simulink model "CONTROL_SYSTEM_V3"  (R2024a)
settings: Solver=FixedStepAuto  StartTime=0.0  StopTime=inf  FixedStep=0.01  RelTol=1e-3
values from neighbouring files (symbols this model uses):
  Beta1 = 3*Omega_o    (= 15)    [CONTROL_SYSTEM_VAR.m]
  Beta2 = 3*(Omega_o^2)    (= 75)    [CONTROL_SYSTEM_VAR.m]
  Beta3 = (Omega_o^3)    (= 125)    [CONTROL_SYSTEM_VAR.m]
  Desire_Max = 255    [CONTROL_SYSTEM_VAR.m]
  Desire_Min = 0    [CONTROL_SYSTEM_VAR.m]
  Direction_Pin = 1    [CONTROL_SYSTEM_VAR.m]
  EN_Pin = 0    [CONTROL_SYSTEM_VAR.m]
  J_aet = 0.0035    [CONTROL_SYSTEM_VAR.m]
  Kd = 2    [CONTROL_SYSTEM_VAR.m]
  Ki = 4    [CONTROL_SYSTEM_VAR.m]
  Kn = 0.1    [CONTROL_SYSTEM_VAR.m]
  Kp = 1.4    [CONTROL_SYSTEM_VAR.m]
  omga_c = 10    [CONTROL_SYSTEM_VAR.m]
  roa = 0.24    [CONTROL_SYSTEM_VAR.m]
undefined symbols (not defined in the file or in its folder): sigbuilder_block
libraries: arduinolib x30, simulink_extras x14, simulink x5, slpidlib x4, SignalEditorBlockLib x3, slctrl_adaptive x2, spsOnDelayLib x2, slctrl_autotuning x2
(part 2 of 5)

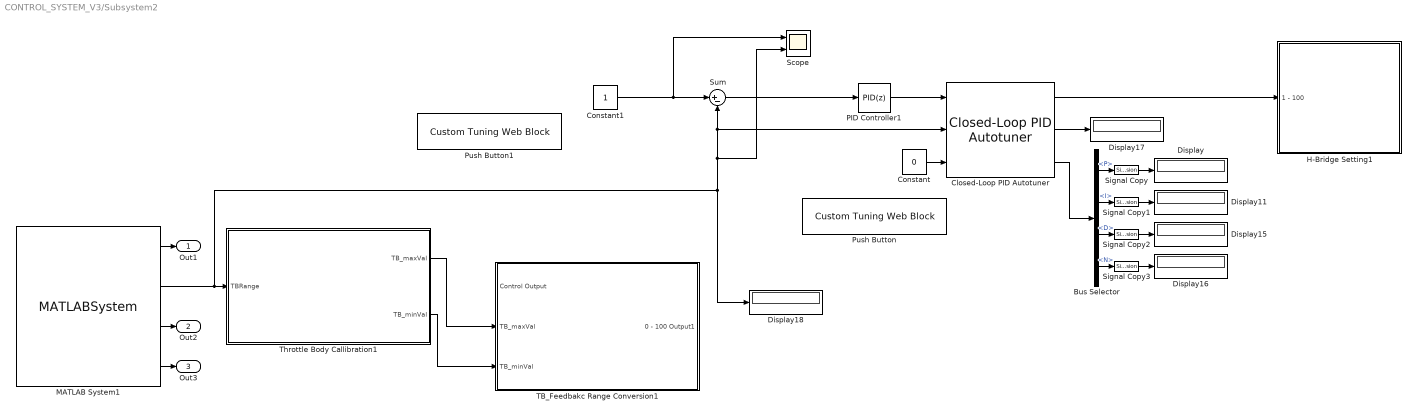
== system CONTROL_SYSTEM_V3/Subsystem2 ==
  Bus Selector : BusSelector  OutputSignals=P,I,D,N
  Closed-Loop PID Autotuner : slctrl_autotuning/Closed-Loop PID Autotuner  PIDType=PID  PIDForm=Parallel  TimeDomain=discrete-time  DiscreteTs=0.1  TuningTs=0.2  UseTuningTs=off  IntegratorFormula=Forward Euler  FilterFormula=Forward Euler  ContinuousTs=-1  Bandwidth=1  UseExternalWC=off  TargetPM=60  UseExternalPM=off  UseExternalAchievedPM=off  ExperimentMode=Superposition  PlantType=Stable  PlantSign=Positive  AmpSine=1  UseExternalAmpSine=off  UseExternalFRD=off  UseExternalU0=off  UseCompanion=off  NotDeployTuningModule=off  UsePLCCoder=off  OutputMode=control action + perturbation  BlockDataType=double  UseConnectedPID=on  blockpath=[]  tunedP=0  tunedI=0  tunedD=0  tunedN=100  tunedPM=0  EstimationWindowSize=3  UseExternalTuningParams=off  SingleMultiRateVariant=SingleSamplingRate  NumEstimationPeriods=4  NumSettlingPeriods=2  NumOfPRBSPeriod=1  PRBSSignalOrder=12  ExperimentModeVariant=VariantSuperimposed  OutputChoice=VariantCandD
      settings: LibrarySourceBlock=slctrlblks/Autotuning/Closed-Loop PID Autotuner
  Constant : Constant  Value=0
  Constant1 : Constant
  Display{,11,15..18} (6 alike) : Display
  H-Bridge Setting1 : Subsystem
      mask Display: image('H-Bridge.JPG');
  MATLAB System1 : MATLABSystem  System=ADS1115_Vread  SetGain=int16( 16 )  SampleTime=-1
      mask Type: ADS1115_Vread
      mask Display:
      | color('white');plot([100,100,100,100]*1,[100,100,100,100]*1);plot([100,100,100,100]*0,[100,100,100,100]*0);color('blue');text(38, 92, 'IO Device Builder','horizontalAlignment', 'right');
      | color('black');text(52,50,' ADS1115_Vread','horizontalAlignment','center');
      | port_label('output',1,'V0');port_label('output',2,'V1');port_label('output',3,'V2');port_label('output',4,'V3');
  PID Controller1 : slpidlib/PID Controller  Controller=PID  Form=Parallel  TimeDomain=Discrete-time  UseExternalTs=off  SampleTime=-1  IntegratorMethod=Forward Euler  FilterMethod=Forward Euler  ControllerParametersSource=internal  P=0  I=185.8371  UseKiTs=off  D=87.2762  UseExternalDerivativeSource=off  N=100  UseFilter=on  TunerSelectOption=Transfer Function Based (PID Tuner App)  InitialConditionSource=internal  InitialConditionForIntegrator=0  InitialConditionForFilter=0  DifferentiatorICPrevScaledInput=0  ExternalReset=none  TrackingMode=off  Kt=1  LimitOutput=off  SatLimitsSource=internal  UpperSaturationLimit=inf  LowerSaturationLimit=-inf  LinearizeAsGain=on  AntiWindupMode=none  Kb=1  LimitIntegrator=off  UpperIntegratorSaturationLimit=inf  LowerIntegratorSaturationLimit=-inf  POutMin=[]  POutMax=[]  IOutMin=[]  IOutMax=[]  DOutMin=[]  DOutMax=[]  NOutMin=[]  NOutMax=[]  SumOutMin=[]  SumOutMax=[]  SaturationOutMin=[]  SaturationOutMax=[]  PParamMin=[]  PParamMax=[]  IParamMin=[]  IParamMax=[]  DParamMin=[]  DParamMax=[]  NParamMin=[]  NParamMax=[]  KbParamMin=[]  KbParamMax=[]  KtParamMin=[]  KtParamMax=[]  KbOutMin=[]  KbOutMax=[]  KtOutMin=[]  KtOutMax=[]  IntegratorOutMin=[]  IntegratorOutMax=[]  FilterOutMin=[]  FilterOutMax=[]  SumI1OutMin=[]  SumI1OutMax=[]  SumI2OutMin=[]  SumI2OutMax=[]  SumI3OutMin=[]  SumI3OutMax=[]  SumI4OutMin=[]  SumI4OutMax=[]  SumDOutMin=[]  SumDOutMax=[]  DifferentiatorOutMin=[]  DifferentiatorOutMax=[]  FilterDiffOutCoefMin=[]  FilterDiffOutCoefMax=[]  ReciprocalOutMin=[]  ReciprocalOutMax=[]  SumDenOutMin=[]  SumDenOutMax=[]  SumNumOutMin=[]  SumNumOutMax=[]  DivideOutMin=[]  DivideOutMax=[]  UdiffTsProdOutMin=[]  UdiffTsProdOutMax=[]  NTsProdOutMin=[]  NTsProdOutMax=[]  UintegralTsProdOutMin=[]  UintegralTsProdOutMax=[]  UngainTsProdOutMin=[]  UngainTsProdOutMax=[]  ClampingZeroOutDataTypeStr=Inherit: Inherit via back propagation  ClampingZeroOutMin=[]  ClampingZeroOutMax=[]  FilterDenConstantOutDataTypeStr=Inherit: Inherit via back propagation  FilterDenConstantOutMin=[]  FilterDenConstantOutMax=[]  PCopyOutDataTypeStr=Inherit: Inherit via back propagation  PCopyOutMin=[]  PCopyOutMax=[]  NCopyOutDataTypeStr=Inherit: Inherit via back propagation  NCopyOutMin=[]  NCopyOutMax=[]  IntegratorContinuousStateAttributes=''  IntegratorStateMustResolveToSignalObject=off  IntegratorRTWStateStorageClass=Auto  FilterContinuousStateAttributes=''  FilterStateMustResolveToSignalObject=off  FilterRTWStateStorageClass=Auto  ParallelPVariant=InternalParameters  IdealPVariant=Disabled  IVariant=InternalParameters  DVariant=InternalParameters  IntegratorVariant=Discrete  SatVariant=Disabled  AWVariant=Passthrough  PCopyVariant=Disabled  TRVariant=Disabled  FdbkBlocksVariant=Forward  IdealPFdbkVariant=Disabled  SatFdbkVariant=Disabled  DerivativeFilterVariant=ForwardEulerFilter  NVariant=InternalParameters  NCopyVariant=Disabled  FilterICVariant=InternalICsFilter  IntegratorICVariant=InternalICs  ExternalResetVariant=Disabled  TRSumVariant=Passthrough  SumFdbkVariant=Disabled  SumVariant=Sum_PID  TsampFilterVariant=InternalTs  TsampNgainVariant=Passthrough  TsampIntegralVariant=Disabled_SignalSpec  ExternalSaturationOutDataTypeStr=Inherit: Same as second input  DerivativeSourceVariant=ErrorSignal
  Push Button : CustomTuningWebBlock  LabelPosition=Hide  ShowInitialText=on  Configuration="{\"components\":[{\"name\":\"BackgroundImageComponent\",\"settings\":{\"image\":{\"size\":[0,0],\"src\":\"default\",\"srcOrientation\":\"horizontal\"},\"position\":[0,0,1,1],\"scaleMode\":\"0\"}},{\"name\":\"ButtonStateComponent\",\"settings\":{\"buttonType\":\"latch\",\"clickFcn\":\"\",\"image\":{\"size\":[180,45],\"srcOrientation\":\"Right\"},\"latched\":false,\"offValue\":null,\"onValue\":\"1\",\"position\":[0,0,1,1],\"pressDelay\":\"500\",\"pressFcn\":\"\",\"repeatInterval\":\"0\",\"states\":[{\"horizontalAlignment\":\"center\",\"image\":{\"position\":[0.04444444444444445,0.005555555555555536,0.9888888888888889,0.9111111111111111],\"size\":[0.9888888888888889,0.9111111111111111],\"src\":\"data:image\\/svg+xml;base64,PHN2ZyB4bWxucz0iaHR0cDovL3d3dy53My5vcmcvMjAwMC9zdmciIHhtbG5zOnhsaW5rPSJodHRwOi8vd3d3LnczLm9yZy8xOTk5L3hsaW5rIiB2aWV3Qm94PSIwIDAgMTc3LjI1IDQwLjg4Ij48ZGVmcz48c3R5bGU+LmNscy0xe2ZpbGw6dXJsKCNyYWRpYWwtZ3JhZGllbnQpO30uY2xzLTJ7ZmlsbDp1cmwoI2xpbmVhci1ncmFkaWVudCk7fS5jbHMtM3tmaWxsOnVybCgjbGluZWFyLWdyYWRpZW50LTIpO308L3N0eWxlPjxyYWRpYWxHcmFkaWVudCBpZD0icmFkaWFsLWdyYWRpZW50IiBjeD0iOTAuMDkiIGN5PSIyMi42NiIgcj0i ...(+2212 chars)\",\"srcOrientation\":\"Right\"},\"label\":{\"color\":[1,1,0.78,1],\"icon\":{\"size\":[0.1,0.375],\"src\":\"data:image\\/svg+xml;base64,PHN2ZyBpZD0iT2ZmIiB4bWxucz0iaHR0cDovL3d3dy53My5vcmcvMjAwMC9zdmciIHhtbG5zOnhsaW5rPSJodHRwOi8vd3d3LnczLm9yZy8xOTk5L3hsaW5rIiB2aWV3Qm94PSIwIDAgNTAgNTAiPjxkZWZzPjxzdHlsZT4uY2xzLTF7ZmlsbDojN2Y4MDgwO3N0cm9rZTojMjcyNjI2O3N0cm9rZS1taXRlcmxpbWl0OjEwO3N0cm9rZS13aWR0aDozcHg7fS5jbHMtMntmaWxsOnVybCgjbGluZWFyLWdyYWRpZW50KTt9PC9zdHlsZT48bGluZWFyR3JhZGllbnQgaWQ9ImxpbmVhci1ncmFkaWVudCIgeDE9IjI1IiB5MT0iOSIgeDI9IjI1IiB5Mj0iMzciIGdyYWRpZW50VW5pdHM9InVzZXJTcGFjZU9uVXNlIj48c3RvcCBvZmZzZXQ9IjAiIHN0b3AtY29sb3I9IiNmZmYiIHN0b3Atb3BhY2l0eT0iMC43NSIvPjxzdG9wIG9mZnNldD0iMSIgc3RvcC1jb2xvcj0iI2ZmZiIgc3RvcC1vcGFjaXR5PSIwIi8+PC9saW5lYXJHcmFkaWVudD48L2RlZnM+PGNpcmNsZSBjbGFzcz0iY2xzLTEiIGN4PSIyNSIgY3k9IjI1IiByPSIyMCIvPjxjaXJjbGUgY2xhc3M9ImNscy0yIiBjeD0iMjUiIGN5PSIyMyIgcj0iMTQiLz48L3N2Zz4=\",\"srcOrientation\":\"Right\"},\"iconPlacement\":\"left\",\"opacity\":1,\"show\":true,\"text\":{\"content\":\"Button\",\"font\":\"Helvetica\",\"fontSize\":14}},\"labelOffset\":[0,0],\"verticalAlignment\":\"middle\"},{\"horizontalAlignment\":\"center\",\"image\":{\"position\":[0.04444444444444445,0.005555555555555536,0.9888888888888889,0.9111111111111111],\"size\":[0.9888888888888889,0.9111111111111111],\"src\":\"data:image\\/svg+xml;base64,PHN2ZyB4bWxucz0iaHR0cDovL3d3dy53My5vcmcvMjAwMC9zdmciIHhtbG5zOnhsaW5rPSJodHRwOi8vd3d3LnczLm9yZy8xOTk5L3hsaW5rIiB2aWV3Qm94PSIwIDAgMTc3LjI1IDQwLjg4Ij48ZGVmcz48c3R5bGU+LmNscy0xe2ZpbGw6dXJsKCNyYWRpYWwtZ3JhZGllbnQpO30uY2xzLTJ7ZmlsbDp1cmwoI2xpbmVhci1ncmFkaWVudCk7fS5jbHMtM3tmaWxsOnVybCgjbGluZWFyLWdyYWRpZW50LTIpO308L3N0eWxlPjxyYWRpYWxHcmFkaWVudCBpZD0icmFkaWFsLWdyYWRpZW50IiBjeD0iOTAuMDkiIGN5PSIyMi42NiIgcj0i ...(+2216 chars)\",\"srcOrientation\":\"Right\"},\"label\":{\"color\":[1,1,0.78,1],\"icon\":{\"size\":[0.1,0.375],\"src\":\"data:image\\/svg+xml;base64,PHN2ZyB4bWxucz0iaHR0cDovL3d3dy53My5vcmcvMjAwMC9zdmciIHhtbG5zOnhsaW5rPSJodHRwOi8vd3d3LnczLm9yZy8xOTk5L3hsaW5rIiB2aWV3Qm94PSIwIDAgNTAgNTAiPjxkZWZzPjxzdHlsZT4uY2xzLTF7ZmlsbDojNmFiZDQ1O3N0cm9rZTojMjcyNjI2O3N0cm9rZS1taXRlcmxpbWl0OjEwO3N0cm9rZS13aWR0aDozcHg7fS5jbHMtMntmaWxsOnVybCgjbGluZWFyLWdyYWRpZW50KTt9PC9zdHlsZT48bGluZWFyR3JhZGllbnQgaWQ9ImxpbmVhci1ncmFkaWVudCIgeDE9IjI1IiB5MT0iOSIgeDI9IjI1IiB5Mj0iMzciIGdyYWRpZW50VW5pdHM9InVzZXJTcGFjZU9uVXNlIj48c3RvcCBvZmZzZXQ9IjAiIHN0b3AtY29sb3I9IiNmZmYiIHN0b3Atb3BhY2l0eT0iMC43NSIvPjxzdG9wIG9mZnNldD0iMSIgc3RvcC1jb2xvcj0iI2ZmZiIgc3RvcC1vcGFjaXR5PSIwIi8+PC9saW5lYXJHcmFkaWVudD48L2RlZnM+PGcgaWQ9Ik9uIj48Y2lyY2xlIGNsYXNzPSJjbHMtMSIgY3g9IjI1IiBjeT0iMjUiIHI9IjIwIi8+PGNpcmNsZSBjbGFzcz0iY2xzLTIiIGN4PSIyNSIgY3k9IjIzIiByPSIxNCIvPjwvZz48L3N2Zz4=\",\"srcOrientation\":\"Right\"},\"iconPlacement\":\"left\",\"opacity\":1,\"show\":true,\"text\":{\"content\":\"Button\",\"font\":\"Helvetica\",\"fontSize\":14}},\"labelOffset\":[0.025,0],\"verticalAlignment\":\"middle\"},{\"horizontalAlignment\":\"center\",\"image\":{\"position\":[0.04444444444444445,0.005555555555555536,0.9888888888888889,0.9111111111111111],\"size\":[0.9888888888888889,0.9111111111111111],\"src\":\"data:image\\/svg+xml;base64,PHN2ZyB4bWxucz0iaHR0cDovL3d3dy53My5vcmcvMjAwMC9zdmciIHhtbG5zOnhsaW5rPSJodHRwOi8vd3d3LnczLm9yZy8xOTk5L3hsaW5rIiB2aWV3Qm94PSIwIDAgMTc3LjI1IDQwLjg4Ij48ZGVmcz48c3R5bGU+LmNscy0xe2ZpbGw6dXJsKCNyYWRpYWwtZ3JhZGllbnQpO30uY2xzLTJ7ZmlsbDp1cmwoI2xpbmVhci1ncmFkaWVudCk7fS5jbHMtM3tmaWxsOnVybCgjbGluZWFyLWdyYWRpZW50LTIpO308L3N0eWxlPjxyYWRpYWxHcmFkaWVudCBpZD0icmFkaWFsLWdyYWRpZW50IiBjeD0iOTAuMDkiIGN5PSIyMi42NiIgcj0i ...(+2212 chars)\",\"srcOrientation\":\"Right\"},\"label\":{\"color\":[1,1,0.78,1],\"icon\":{\"size\":[0.1,0.375],\"src\":\"data:image\\/svg+xml;base64,PHN2ZyB4bWxucz0iaHR0cDovL3d3dy53My5vcmcvMjAwMC9zdmciIHhtbG5zOnhsaW5rPSJodHRwOi8vd3d3LnczLm9yZy8xOTk5L3hsaW5rIiB2aWV3Qm94PSIwIDAgNTAgNTAiPjxkZWZzPjxzdHlsZT4uY2xzLTF7ZmlsbDojNmFiZDQ1O3N0cm9rZTojMjcyNjI2O3N0cm9rZS1taXRlcmxpbWl0OjEwO3N0cm9rZS13aWR0aDozcHg7fS5jbHMtMntmaWxsOnVybCgjbGluZWFyLWdyYWRpZW50KTt9PC9zdHlsZT48bGluZWFyR3JhZGllbnQgaWQ9ImxpbmVhci1ncmFkaWVudCIgeDE9IjI1IiB5MT0iOSIgeDI9IjI1IiB5Mj0iMzciIGdyYWRpZW50VW5pdHM9InVzZXJTcGFjZU9uVXNlIj48c3RvcCBvZmZzZXQ9IjAiIHN0b3AtY29sb3I9IiNmZmYiIHN0b3Atb3BhY2l0eT0iMC43NSIvPjxzdG9wIG9mZnNldD0iMSIgc3RvcC1jb2xvcj0iI2ZmZiIgc3RvcC1vcGFjaXR5PSIwIi8+PC9saW5lYXJHcmFkaWVudD48L2RlZnM+PGcgaWQ9Ik9uIj48Y2lyY2xlIGNsYXNzPSJjbHMtMSIgY3g9IjI1IiBjeT0iMjUiIHI9IjIwIi8+PGNpcmNsZSBjbGFzcz0iY2xzLTIiIGN4PSIyNSIgY3k9IjIzIiByPSIxNCIvPjwvZz48L3N2Zz4=\",\"srcOrientation\":\"Right\"},\"iconPlacement\":\"left\",\"opacity\":1,\"show\":true,\"text\":{\"content\":\"Button\",\"font\":\"Helvetica\",\"fontSize\":14}},\"labelOffset\":[0,0],\"verticalAlignment\":\"middle\"},{\"horizontalAlignment\":\"center\",\"image\":{\"position\":[0.04444444444444445,0.005555555555555536,0.9888888888888889,0.9111111111111111],\"size\":[0.9888888888888889,0.9111111111111111],\"src\":\"data:image\\/svg+xml;base64,PHN2ZyB4bWxucz0iaHR0cDovL3d3dy53My5vcmcvMjAwMC9zdmciIHhtbG5zOnhsaW5rPSJodHRwOi8vd3d3LnczLm9yZy8xOTk5L3hsaW5rIiB2aWV3Qm94PSIwIDAgMTc3LjI1IDQwLjg4Ij48ZGVmcz48c3R5bGU+LmNscy0xe2ZpbGw6dXJsKCNyYWRpYWwtZ3JhZGllbnQpO30uY2xzLTJ7ZmlsbDp1cmwoI2xpbmVhci1ncmFkaWVudCk7fS5jbHMtM3tmaWxsOnVybCgjbGluZWFyLWdyYWRpZW50LTIpO308L3N0eWxlPjxyYWRpYWxHcmFkaWVudCBpZD0icmFkaWFsLWdyYWRpZW50IiBjeD0iOTAuMDkiIGN5PSIyMi42NiIgcj0i ...(+2216 chars)\",\"srcOrientation\":\"Right\"},\"label\":{\"color\":[1,1,0.78,1],\"icon\":{\"size\":[0.1,0.375],\"src\":\"data:image\\/svg+xml;base64,PHN2ZyBpZD0iT2ZmIiB4bWxucz0iaHR0cDovL3d3dy53My5vcmcvMjAwMC9zdmciIHhtbG5zOnhsaW5rPSJodHRwOi8vd3d3LnczLm9yZy8xOTk5L3hsaW5rIiB2aWV3Qm94PSIwIDAgNTAgNTAiPjxkZWZzPjxzdHlsZT4uY2xzLTF7ZmlsbDojN2Y4MDgwO3N0cm9rZTojMjcyNjI2O3N0cm9rZS1taXRlcmxpbWl0OjEwO3N0cm9rZS13aWR0aDozcHg7fS5jbHMtMntmaWxsOnVybCgjbGluZWFyLWdyYWRpZW50KTt9PC9zdHlsZT48bGluZWFyR3JhZGllbnQgaWQ9ImxpbmVhci1ncmFkaWVudCIgeDE9IjI1IiB5MT0iOSIgeDI9IjI1IiB5Mj0iMzciIGdyYWRpZW50VW5pdHM9InVzZXJTcGFjZU9uVXNlIj48c3RvcCBvZmZzZXQ9IjAiIHN0b3AtY29sb3I9IiNmZmYiIHN0b3Atb3BhY2l0eT0iMC43NSIvPjxzdG9wIG9mZnNldD0iMSIgc3RvcC1jb2xvcj0iI2ZmZiIgc3RvcC1vcGFjaXR5PSIwIi8+PC9saW5lYXJHcmFkaWVudD48L2RlZnM+PGNpcmNsZSBjbGFzcz0iY2xzLTEiIGN4PSIyNSIgY3k9IjI1IiByPSIyMCIvPjxjaXJjbGUgY2xhc3M9ImNscy0yIiBjeD0iMjUiIGN5PSIyMyIgcj0iMTQiLz48L3N2Zz4=\",\"srcOrientation\":\"Right\"},\"iconPlacement\":\"left\",\"opacity\":1,\"show\":true,\"text\":{\"content\":\"Button\",\"font\":\"Helvetica\",\"fontSize\":14}},\"labelOffset\":[0.025,0],\"verticalAlignment\":\"middle\"}]}},{\"name\":\"ForegroundImageComponent\",\"settings\":{\"image\":{\"size\":[0,0],\"src\":\"default\",\"srcOrientation\":\"horizontal\"},\"isForeground\":1,\"position\":[0,0,1,1],\"scaleMode\":\"0\"}}],\"settings\":{\"BindingType\":\"param\",\"aspectRatio\":3.7777777777777777,\"backgroundColor\":[0,0,0,\"1\"],\"backgroundOffset\":0,\"backgroundOpacity\":1,\"fixedAspectRatio\":\"on\",\"foregroundColor\":[252,252,196],\"showBackgroundColor\":false,\"variant\":\"push\",\"version\":\"R2023a\"},\"type\":\"Button\"}"
  Push Button1 : CustomTuningWebBlock  LabelPosition=Hide  ShowInitialText=on  Configuration="{\"components\":[{\"name\":\"BackgroundImageComponent\",\"settings\":{\"image\":{\"size\":[0,0],\"src\":\"default\",\"srcOrientation\":\"horizontal\"},\"position\":[0,0,1,1],\"scaleMode\":\"0\"}},{\"name\":\"ButtonStateComponent\",\"settings\":{\"buttonType\":\"latch\",\"clickFcn\":\"\",\"image\":{\"size\":[180,45],\"srcOrientation\":\"Right\"},\"latched\":true,\"offValue\":0,\"onValue\":\"1\",\"position\":[0,0,1,1],\"pressDelay\":\"500\",\"pressFcn\":\"\",\"repeatInterval\":\"0\",\"states\":[{\"horizontalAlignment\":\"center\",\"image\":{\"position\":[0.04444444444444445,0.005555555555555536,0.9888888888888889,0.9111111111111111],\"size\":[0.9888888888888889,0.9111111111111111],\"src\":\"data:image\\/svg+xml;base64,PHN2ZyB4bWxucz0iaHR0cDovL3d3dy53My5vcmcvMjAwMC9zdmciIHhtbG5zOnhsaW5rPSJodHRwOi8vd3d3LnczLm9yZy8xOTk5L3hsaW5rIiB2aWV3Qm94PSIwIDAgMTc3LjI1IDQwLjg4Ij48ZGVmcz48c3R5bGU+LmNscy0xe2ZpbGw6dXJsKCNyYWRpYWwtZ3JhZGllbnQpO30uY2xzLTJ7ZmlsbDp1cmwoI2xpbmVhci1ncmFkaWVudCk7fS5jbHMtM3tmaWxsOnVybCgjbGluZWFyLWdyYWRpZW50LTIpO308L3N0eWxlPjxyYWRpYWxHcmFkaWVudCBpZD0icmFkaWFsLWdyYWRpZW50IiBjeD0iOTAuMDkiIGN5PSIyMi42NiIgcj0i ...(+2212 chars)\",\"srcOrientation\":\"Right\"},\"label\":{\"color\":[1,1,0.78,1],\"icon\":{\"size\":[0.1,0.375],\"src\":\"data:image\\/svg+xml;base64,PHN2ZyBpZD0iT2ZmIiB4bWxucz0iaHR0cDovL3d3dy53My5vcmcvMjAwMC9zdmciIHhtbG5zOnhsaW5rPSJodHRwOi8vd3d3LnczLm9yZy8xOTk5L3hsaW5rIiB2aWV3Qm94PSIwIDAgNTAgNTAiPjxkZWZzPjxzdHlsZT4uY2xzLTF7ZmlsbDojN2Y4MDgwO3N0cm9rZTojMjcyNjI2O3N0cm9rZS1taXRlcmxpbWl0OjEwO3N0cm9rZS13aWR0aDozcHg7fS5jbHMtMntmaWxsOnVybCgjbGluZWFyLWdyYWRpZW50KTt9PC9zdHlsZT48bGluZWFyR3JhZGllbnQgaWQ9ImxpbmVhci1ncmFkaWVudCIgeDE9IjI1IiB5MT0iOSIgeDI9IjI1IiB5Mj0iMzciIGdyYWRpZW50VW5pdHM9InVzZXJTcGFjZU9uVXNlIj48c3RvcCBvZmZzZXQ9IjAiIHN0b3AtY29sb3I9IiNmZmYiIHN0b3Atb3BhY2l0eT0iMC43NSIvPjxzdG9wIG9mZnNldD0iMSIgc3RvcC1jb2xvcj0iI2ZmZiIgc3RvcC1vcGFjaXR5PSIwIi8+PC9saW5lYXJHcmFkaWVudD48L2RlZnM+PGNpcmNsZSBjbGFzcz0iY2xzLTEiIGN4PSIyNSIgY3k9IjI1IiByPSIyMCIvPjxjaXJjbGUgY2xhc3M9ImNscy0yIiBjeD0iMjUiIGN5PSIyMyIgcj0iMTQiLz48L3N2Zz4=\",\"srcOrientation\":\"Right\"},\"iconPlacement\":\"left\",\"opacity\":1,\"show\":true,\"text\":{\"content\":\"Button\",\"font\":\"Helvetica\",\"fontSize\":14}},\"labelOffset\":[0,0],\"verticalAlignment\":\"middle\"},{\"horizontalAlignment\":\"center\",\"image\":{\"position\":[0.04444444444444445,0.005555555555555536,0.9888888888888889,0.9111111111111111],\"size\":[0.9888888888888889,0.9111111111111111],\"src\":\"data:image\\/svg+xml;base64,PHN2ZyB4bWxucz0iaHR0cDovL3d3dy53My5vcmcvMjAwMC9zdmciIHhtbG5zOnhsaW5rPSJodHRwOi8vd3d3LnczLm9yZy8xOTk5L3hsaW5rIiB2aWV3Qm94PSIwIDAgMTc3LjI1IDQwLjg4Ij48ZGVmcz48c3R5bGU+LmNscy0xe2ZpbGw6dXJsKCNyYWRpYWwtZ3JhZGllbnQpO30uY2xzLTJ7ZmlsbDp1cmwoI2xpbmVhci1ncmFkaWVudCk7fS5jbHMtM3tmaWxsOnVybCgjbGluZWFyLWdyYWRpZW50LTIpO308L3N0eWxlPjxyYWRpYWxHcmFkaWVudCBpZD0icmFkaWFsLWdyYWRpZW50IiBjeD0iOTAuMDkiIGN5PSIyMi42NiIgcj0i ...(+2216 chars)\",\"srcOrientation\":\"Right\"},\"label\":{\"color\":[1,1,0.78,1],\"icon\":{\"size\":[0.1,0.375],\"src\":\"data:image\\/svg+xml;base64,PHN2ZyB4bWxucz0iaHR0cDovL3d3dy53My5vcmcvMjAwMC9zdmciIHhtbG5zOnhsaW5rPSJodHRwOi8vd3d3LnczLm9yZy8xOTk5L3hsaW5rIiB2aWV3Qm94PSIwIDAgNTAgNTAiPjxkZWZzPjxzdHlsZT4uY2xzLTF7ZmlsbDojNmFiZDQ1O3N0cm9rZTojMjcyNjI2O3N0cm9rZS1taXRlcmxpbWl0OjEwO3N0cm9rZS13aWR0aDozcHg7fS5jbHMtMntmaWxsOnVybCgjbGluZWFyLWdyYWRpZW50KTt9PC9zdHlsZT48bGluZWFyR3JhZGllbnQgaWQ9ImxpbmVhci1ncmFkaWVudCIgeDE9IjI1IiB5MT0iOSIgeDI9IjI1IiB5Mj0iMzciIGdyYWRpZW50VW5pdHM9InVzZXJTcGFjZU9uVXNlIj48c3RvcCBvZmZzZXQ9IjAiIHN0b3AtY29sb3I9IiNmZmYiIHN0b3Atb3BhY2l0eT0iMC43NSIvPjxzdG9wIG9mZnNldD0iMSIgc3RvcC1jb2xvcj0iI2ZmZiIgc3RvcC1vcGFjaXR5PSIwIi8+PC9saW5lYXJHcmFkaWVudD48L2RlZnM+PGcgaWQ9Ik9uIj48Y2lyY2xlIGNsYXNzPSJjbHMtMSIgY3g9IjI1IiBjeT0iMjUiIHI9IjIwIi8+PGNpcmNsZSBjbGFzcz0iY2xzLTIiIGN4PSIyNSIgY3k9IjIzIiByPSIxNCIvPjwvZz48L3N2Zz4=\",\"srcOrientation\":\"Right\"},\"iconPlacement\":\"left\",\"opacity\":1,\"show\":true,\"text\":{\"content\":\"Button\",\"font\":\"Helvetica\",\"fontSize\":14}},\"labelOffset\":[0.025,0],\"verticalAlignment\":\"middle\"},{\"horizontalAlignment\":\"center\",\"image\":{\"position\":[0.04444444444444445,0.005555555555555536,0.9888888888888889,0.9111111111111111],\"size\":[0.9888888888888889,0.9111111111111111],\"src\":\"data:image\\/svg+xml;base64,PHN2ZyB4bWxucz0iaHR0cDovL3d3dy53My5vcmcvMjAwMC9zdmciIHhtbG5zOnhsaW5rPSJodHRwOi8vd3d3LnczLm9yZy8xOTk5L3hsaW5rIiB2aWV3Qm94PSIwIDAgMTc3LjI1IDQwLjg4Ij48ZGVmcz48c3R5bGU+LmNscy0xe2ZpbGw6dXJsKCNyYWRpYWwtZ3JhZGllbnQpO30uY2xzLTJ7ZmlsbDp1cmwoI2xpbmVhci1ncmFkaWVudCk7fS5jbHMtM3tmaWxsOnVybCgjbGluZWFyLWdyYWRpZW50LTIpO308L3N0eWxlPjxyYWRpYWxHcmFkaWVudCBpZD0icmFkaWFsLWdyYWRpZW50IiBjeD0iOTAuMDkiIGN5PSIyMi42NiIgcj0i ...(+2212 chars)\",\"srcOrientation\":\"Right\"},\"label\":{\"color\":[1,1,0.78,1],\"icon\":{\"size\":[0.1,0.375],\"src\":\"data:image\\/svg+xml;base64,PHN2ZyB4bWxucz0iaHR0cDovL3d3dy53My5vcmcvMjAwMC9zdmciIHhtbG5zOnhsaW5rPSJodHRwOi8vd3d3LnczLm9yZy8xOTk5L3hsaW5rIiB2aWV3Qm94PSIwIDAgNTAgNTAiPjxkZWZzPjxzdHlsZT4uY2xzLTF7ZmlsbDojNmFiZDQ1O3N0cm9rZTojMjcyNjI2O3N0cm9rZS1taXRlcmxpbWl0OjEwO3N0cm9rZS13aWR0aDozcHg7fS5jbHMtMntmaWxsOnVybCgjbGluZWFyLWdyYWRpZW50KTt9PC9zdHlsZT48bGluZWFyR3JhZGllbnQgaWQ9ImxpbmVhci1ncmFkaWVudCIgeDE9IjI1IiB5MT0iOSIgeDI9IjI1IiB5Mj0iMzciIGdyYWRpZW50VW5pdHM9InVzZXJTcGFjZU9uVXNlIj48c3RvcCBvZmZzZXQ9IjAiIHN0b3AtY29sb3I9IiNmZmYiIHN0b3Atb3BhY2l0eT0iMC43NSIvPjxzdG9wIG9mZnNldD0iMSIgc3RvcC1jb2xvcj0iI2ZmZiIgc3RvcC1vcGFjaXR5PSIwIi8+PC9saW5lYXJHcmFkaWVudD48L2RlZnM+PGcgaWQ9Ik9uIj48Y2lyY2xlIGNsYXNzPSJjbHMtMSIgY3g9IjI1IiBjeT0iMjUiIHI9IjIwIi8+PGNpcmNsZSBjbGFzcz0iY2xzLTIiIGN4PSIyNSIgY3k9IjIzIiByPSIxNCIvPjwvZz48L3N2Zz4=\",\"srcOrientation\":\"Right\"},\"iconPlacement\":\"left\",\"opacity\":1,\"show\":true,\"text\":{\"content\":\"Button\",\"font\":\"Helvetica\",\"fontSize\":14}},\"labelOffset\":[0,0],\"verticalAlignment\":\"middle\"},{\"horizontalAlignment\":\"center\",\"image\":{\"position\":[0.04444444444444445,0.005555555555555536,0.9888888888888889,0.9111111111111111],\"size\":[0.9888888888888889,0.9111111111111111],\"src\":\"data:image\\/svg+xml;base64,PHN2ZyB4bWxucz0iaHR0cDovL3d3dy53My5vcmcvMjAwMC9zdmciIHhtbG5zOnhsaW5rPSJodHRwOi8vd3d3LnczLm9yZy8xOTk5L3hsaW5rIiB2aWV3Qm94PSIwIDAgMTc3LjI1IDQwLjg4Ij48ZGVmcz48c3R5bGU+LmNscy0xe2ZpbGw6dXJsKCNyYWRpYWwtZ3JhZGllbnQpO30uY2xzLTJ7ZmlsbDp1cmwoI2xpbmVhci1ncmFkaWVudCk7fS5jbHMtM3tmaWxsOnVybCgjbGluZWFyLWdyYWRpZW50LTIpO308L3N0eWxlPjxyYWRpYWxHcmFkaWVudCBpZD0icmFkaWFsLWdyYWRpZW50IiBjeD0iOTAuMDkiIGN5PSIyMi42NiIgcj0i ...(+2216 chars)\",\"srcOrientation\":\"Right\"},\"label\":{\"color\":[1,1,0.78,1],\"icon\":{\"size\":[0.1,0.375],\"src\":\"data:image\\/svg+xml;base64,PHN2ZyBpZD0iT2ZmIiB4bWxucz0iaHR0cDovL3d3dy53My5vcmcvMjAwMC9zdmciIHhtbG5zOnhsaW5rPSJodHRwOi8vd3d3LnczLm9yZy8xOTk5L3hsaW5rIiB2aWV3Qm94PSIwIDAgNTAgNTAiPjxkZWZzPjxzdHlsZT4uY2xzLTF7ZmlsbDojN2Y4MDgwO3N0cm9rZTojMjcyNjI2O3N0cm9rZS1taXRlcmxpbWl0OjEwO3N0cm9rZS13aWR0aDozcHg7fS5jbHMtMntmaWxsOnVybCgjbGluZWFyLWdyYWRpZW50KTt9PC9zdHlsZT48bGluZWFyR3JhZGllbnQgaWQ9ImxpbmVhci1ncmFkaWVudCIgeDE9IjI1IiB5MT0iOSIgeDI9IjI1IiB5Mj0iMzciIGdyYWRpZW50VW5pdHM9InVzZXJTcGFjZU9uVXNlIj48c3RvcCBvZmZzZXQ9IjAiIHN0b3AtY29sb3I9IiNmZmYiIHN0b3Atb3BhY2l0eT0iMC43NSIvPjxzdG9wIG9mZnNldD0iMSIgc3RvcC1jb2xvcj0iI2ZmZiIgc3RvcC1vcGFjaXR5PSIwIi8+PC9saW5lYXJHcmFkaWVudD48L2RlZnM+PGNpcmNsZSBjbGFzcz0iY2xzLTEiIGN4PSIyNSIgY3k9IjI1IiByPSIyMCIvPjxjaXJjbGUgY2xhc3M9ImNscy0yIiBjeD0iMjUiIGN5PSIyMyIgcj0iMTQiLz48L3N2Zz4=\",\"srcOrientation\":\"Right\"},\"iconPlacement\":\"left\",\"opacity\":1,\"show\":true,\"text\":{\"content\":\"Button\",\"font\":\"Helvetica\",\"fontSize\":14}},\"labelOffset\":[0.025,0],\"verticalAlignment\":\"middle\"}]}},{\"name\":\"ForegroundImageComponent\",\"settings\":{\"image\":{\"size\":[0,0],\"src\":\"default\",\"srcOrientation\":\"horizontal\"},\"isForeground\":1,\"position\":[0,0,1,1],\"scaleMode\":\"0\"}}],\"settings\":{\"BindingType\":\"param\",\"aspectRatio\":3.7777777777777777,\"backgroundColor\":[0,0,0,\"1\"],\"backgroundOffset\":0,\"backgroundOpacity\":1,\"fixedAspectRatio\":\"on\",\"foregroundColor\":[252,252,196],\"showBackgroundColor\":false,\"variant\":\"push\",\"version\":\"R2023a\"},\"type\":\"Button\"}"
  Scope : Scope  NumInputPorts=2
  Signal Copy{,1..3} (4 alike) : SignalConversion  OverrideOpt=off
  Sum : Sum  Inputs=|+-
  TB_Feedbakc Range Conversion1 : Subsystem
  Throttle Body Callibration1 : MATLAB Function  TreatAsAtomicUnit=on
  Out1 : Outport
  Out2 : Outport  Port=2
  Out3 : Outport  Port=3
  wires:
  Signal Copy/1 -> Display/1
  Closed-Loop PID Autotuner/1 -> H-Bridge Setting1/1(1 - 100)
  Bus Selector/3 -> Signal Copy2/1  "<D>"
  Constant/1 -> Closed-Loop PID Autotuner/3
  MATLAB System1/4 -> Out3/1
  Closed-Loop PID Autotuner/3 -> Bus Selector/1
  MATLAB System1/2 -> Scope/2, Closed-Loop PID Autotuner/2, Sum/2, Display18/1, Throttle Body Callibration1/1(TBRange)
  Closed-Loop PID Autotuner/2 -> Display17/1
  Signal Copy2/1 -> Display15/1
  Bus Selector/4 -> Signal Copy3/1  "<N>"
  Signal Copy1/1 -> Display11/1
  Bus Selector/2 -> Signal Copy1/1  "<I>"
  Bus Selector/1 -> Signal Copy/1  "<P>"
  Signal Copy3/1 -> Display16/1
  Constant1/1 -> Scope/1, Sum/1
  Throttle Body Callibration1/2(TB_minVal) -> TB_Feedbakc Range Conversion1/3(TB_minVal)
  Throttle Body Callibration1/1(TB_maxVal) -> TB_Feedbakc Range Conversion1/2(TB_maxVal)
  PID Controller1/1 -> Closed-Loop PID Autotuner/1
  Sum/1 -> PID Controller1/1
  MATLAB System1/1 -> Out1/1
  MATLAB System1/3 -> Out2/1

== system CONTROL_SYSTEM_V3/Subsystem4 ==
  TBRange : Inport
  Calibration_Input : Inport  Port=2
  PedalRange : Inport  Port=3
  Calibration_Input1 : Inport  Port=4
  Enable : EnablePort
  Pedal Calibration2 : MATLAB Function  TreatAsAtomicUnit=on
  Throttle Body Callibration1 : MATLAB Function  TreatAsAtomicUnit=on
  TB_maxVal : Outport
  TB_minVal : Outport  Port=2
  FP_maxVal : Outport  Port=3
  FP_minVal : Outport  Port=4
  wires:
  Calibration_Input1/1 -> Pedal Calibration2/2(Calibration_Input)
  TBRange/1 -> Throttle Body Callibration1/1(TBRange)
  Throttle Body Callibration1/2(TB_minVal) -> TB_minVal/1
  PedalRange/1 -> Pedal Calibration2/1(PedalRange)
  Pedal Calibration2/2(FP_minVal) -> FP_minVal/1
  Calibration_Input/1 -> Throttle Body Callibration1/2(Calibration_Input)
  Throttle Body Callibration1/1(TB_maxVal) -> TB_maxVal/1
  Pedal Calibration2/1(FP_maxVal) -> FP_maxVal/1
